simulink model "customRestrictionTest"  (R2020b)
settings: Solver=VariableStepAuto  StartTime=0.0  StopTime=10.0  RelTol=1e-3
libraries: fl_lib x6, nesl_utility x4
settings Model: Creator=Edward  LastModifiedBy=Edward

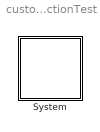
== system customRestrictionTest ==
  System : Subsystem  mask{upstreamPressure=60e5}
      mask prompts: upstreamPressure "Upstream Pressure (Pa)"

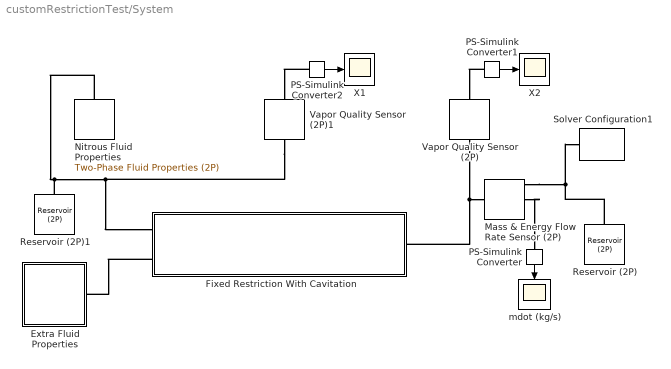
== system customRestrictionTest/System ==
  Extra Fluid Properties : Subsystem  ReferencedSubsystem=nitrousExtraFluidProps
  Fixed Restriction With Cavitation : Subsystem  ReferencedSubsystem=Fixed_Restriction_With_Cavitation  Cv=0.5  x_T=0.3
  Mass & Energy Flow Rate Sensor (2P) : fl_lib/Two-Phase Fluid/Sensors/Mass & Energy Flow Rate Sensor (2P)
      settings: SourceProductBaseCode=SS  InternalSimscapePortConfiguration="{\"Bottom\":[],\"Left\":[{\"id\":\"A\",\"label\":\"A\",\"type\":\"foundation.two_phase_fluid.two_phase_fluid\"}],\"Right\":[{\"id\":\"B\",\"label\":\"B\",\"type\":\"foundation.two_phase_fluid.two_phase_fluid\"},{\"id\":\"M\",\"label\":\"M\",\"type\":\"output\"},{\"id\":\"PHI\",\"label\":\"Phi\",\"type\":\"output\"}],\"Top\":[]}"
  Nitrous Fluid Properties : fl_lib/Two-Phase Fluid/Utilities/Two-Phase Fluid Properties (2P)  u_min=Sim.nitrousFluidTable.u_min kJ/kg  u_max=Sim.nitrousFluidTable.u_max kJ/kg  unorm_liq=Sim.nitrousFluidTable.liquid.unorm  unorm_vap=Sim.nitrousFluidTable.vapor.unorm  p_TLU=Sim.nitrousFluidTable.p MPa  v_liq=Sim.nitrousFluidTable.liquid.v m^3/kg  v_vap=Sim.nitrousFluidTable.vapor.v m^3/kg  s_liq=Sim.nitrousFluidTable.liquid.s kJ/kg/K  s_vap=Sim.nitrousFluidTable.vapor.s kJ/kg/K  T_liq=Sim.nitrousFluidTable.liquid.T K  T_vap=Sim.nitrousFluidTable.vapor.T K  nu_liq=Sim.nitrousFluidTable.liquid.nu mm^2/s  nu_vap=Sim.nitrousFluidTable.vapor.nu mm^2/s  k_liq=Sim.nitrousFluidTable.liquid.k W/(m*K)  k_vap=Sim.nitrousFluidTable.vapor.k W/(m*K)  Pr_liq=Sim.nitrousFluidTable.liquid.Pr  Pr_vap=Sim.nitrousFluidTable.vapor.Pr  u_sat_liq=Sim.nitrousFluidTable.liquid.u_sat kJ/kg  u_sat_vap=Sim.nitrousFluidTable.vapor.u_sat kJ/kg  p_crit=Sim.nitrousFluidTable.p_crit MPa  critical_region=foundation.enum.critical_region.clip  p_crit_fraction=0.12  p_atm=0.101325 MPa  q_rev=0.01 Pa
      settings: SourceProductBaseCode=SS  InternalSimscapePortConfiguration="{\"Bottom\":[],\"Left\":[],\"Right\":[{\"id\":\"A\",\"label\":\"\",\"type\":\"foundation.two_phase_fluid.two_phase_fluid\"}],\"Top\":[]}"
  PS-Simulink Converter : nesl_utility/PS-Simulink Converter  PhysicalDomain=network_engine_domain  SubClassName=ps_output  LeftPortType=input  RightPortType=output  PseudoPeriodic=off  Frequencies=[]  Unit=inherit  AffineConversion=off
  PS-Simulink Converter1 : nesl_utility/PS-Simulink Converter  PhysicalDomain=network_engine_domain  SubClassName=ps_output  LeftPortType=input  RightPortType=output  PseudoPeriodic=off  Frequencies=[]  Unit=inherit  AffineConversion=off
  PS-Simulink Converter2 : nesl_utility/PS-Simulink Converter  PhysicalDomain=network_engine_domain  SubClassName=ps_output  LeftPortType=input  RightPortType=output  PseudoPeriodic=off  Frequencies=[]  Unit=inherit  AffineConversion=off
  Reservoir (2P) : fl_lib/Two-Phase Fluid/Elements/Reservoir (2P)  pressure_spec=foundation.enum.pressure_spec.specified  reservoir_pressure=15e5 Pa  energy_spec=foundation.enum.energy_spec.temperature  reservoir_temperature=293.15 K  reservoir_quality=0.5  reservoir_void_fraction=0.5  reservoir_enthalpy=1500 kJ/kg  reservoir_internal_energy=1500 kJ/kg  area_A=0.01 m^2
      settings: SourceProductBaseCode=SS
  Reservoir (2P)1 : fl_lib/Two-Phase Fluid/Elements/Reservoir (2P)  pressure_spec=foundation.enum.pressure_spec.specified  reservoir_pressure=upstreamPressure Pa  energy_spec=foundation.enum.energy_spec.quality  reservoir_temperature=293.15 K  reservoir_quality=0  reservoir_void_fraction=0.5  reservoir_enthalpy=1500 kJ/kg  reservoir_internal_energy=1500 kJ/kg  area_A=0.01 m^2
      settings: SourceProductBaseCode=SS
  Solver Configuration1 : nesl_utility/Solver Configuration  PhysicalDomain=network_engine_domain  SubClassName=solver  LeftPortType=input  RightPortType=generic  Tones=[]  Harmonics=[]  SimulateNoise=off  Profile=off  UseLocalSampling=off  EnableSwitchedLinearOptims=on  FrequencyDomain=off  UseCCode=off  RelTol=0.001  AbsTol=1e-06  MinStep=1e-09  ToWorkspace=off  RevertToSquareIcSolve=off  NumHomotopyIterations=100  PhasorMode=off  PhasorModeNumHarmonics=1  DoDC=off  ResidualTolerance=1e-9  UseLocalSolver=off  LocalSolverChoice=NE_BACKWARD_EULER_ADVANCER  LocalSolverSampleTime=0.001  DoFixedCost=off  MaxNonlinIter=3  MaxModeIter=2  ComputeImpulses=off  ImpulseIterations=2  LinearAlgebra=auto  EquationFormulation=NE_TIME_EF  DelaysMemoryBudget=1024  AutomaticFiltering=on  FilteringTimeConstant=0.001  PartitionStorageMethod=AS_NEEDED  PartitionMemoryBudget=1024  PartitionMethod=ROBUST
  Vapor Quality Sensor (2P) : fl_lib/Two-Phase Fluid/Sensors/Vapor Quality Sensor (2P)  vapor_fraction_spec=foundation.enum.vapor_fraction_spec.quality
      settings: SourceProductBaseCode=SS  InternalSimscapePortConfiguration="{\"Bottom\":[],\"Left\":[{\"id\":\"A\",\"label\":\"A\",\"type\":\"foundation.two_phase_fluid.two_phase_fluid\"}],\"Right\":[{\"id\":\"X\",\"label\":\"X\",\"type\":\"output\"}],\"Top\":[]}"
  Vapor Quality Sensor (2P)1 : fl_lib/Two-Phase Fluid/Sensors/Vapor Quality Sensor (2P)  vapor_fraction_spec=foundation.enum.vapor_fraction_spec.quality
      settings: SourceProductBaseCode=SS  InternalSimscapePortConfiguration="{\"Bottom\":[],\"Left\":[{\"id\":\"A\",\"label\":\"A\",\"type\":\"foundation.two_phase_fluid.two_phase_fluid\"}],\"Right\":[{\"id\":\"X\",\"label\":\"X\",\"type\":\"output\"}],\"Top\":[]}"
  X1 : Scope
  X2 : Scope
  mdot (kg/s) : Scope
  wires:
  PS-Simulink Converter/1 -> mdot (kg/s)/1
  PS-Simulink Converter1/1 -> X2/1
  PS-Simulink Converter2/1 -> X1/1
  connections:
  Reservoir (2P)/LConn1 -- Mass & Energy Flow Rate Sensor (2P)/RConn1 -- Solver Configuration1/RConn1
  Reservoir (2P)1/LConn1 -- Vapor Quality Sensor (2P)1/LConn1 -- Fixed Restriction With Cavitation/LConn1 -- Nitrous Fluid Properties/RConn1
  Vapor Quality Sensor (2P)/LConn1 -- Fixed Restriction With Cavitation/RConn1 -- Mass & Energy Flow Rate Sensor (2P)/LConn1
  Mass & Energy Flow Rate Sensor (2P)/RConn2 -- PS-Simulink Converter/LConn1
  PS-Simulink Converter1/LConn1 -- Vapor Quality Sensor (2P)/RConn1
  PS-Simulink Converter2/LConn1 -- Vapor Quality Sensor (2P)1/RConn1
  Fixed Restriction With Cavitation/LConn2 -- Extra Fluid Properties/RConn1
